simulink model "MtrCtrl_24V"  (R2023b)
settings: Solver=FixedStepDiscrete  StartTime=0.0  StopTime=1  FixedStep=1e-6  RelTol=1e-3
values from neighbouring files (symbols this model uses):
  B = 0.001889    [MtrCtrl_v01.sldd]    (also in PICal.m = 0.001889; PMSM.m = Simulink.Parameter)
  C_LUT_AngleTable_sng_Null = saveVarsMat.C_LUT_AngleTable_sng_Null    [AngleTable.m]    (also in MtrCtrl_v01.sldd = 0.0015339807878856412 0.0030679615757712823 0.00460194236365; PMSM.m; SinLut.m = sinTable(2,:))
  C_LUT_SinTable_sng_Null = saveVarsMat.C_LUT_SinTable_sng_Null    [AngleTable.m]    (also in MtrCtrl_v01.sldd = 0.0015339801862847655 0.0030679567629659761 0.00460192612044; PMSM.m; SinLut.m = sinTable(1,:))
  C_MATH_OneOverSqrtThree_s32n31_Null = 0.57735026918962584    [MtrCtrl_v01.sldd]    (also in PMSM.m = Simulink.Parameter)
  C_MATH_Pi_u32n30_Null = 3.1415926535897931    [MtrCtrl_v01.sldd]    (also in PMSM.m = Simulink.Parameter)
  C_MATH_SqrtThreeOverThree_s32n31_Null = 0.57735026918962573    [MtrCtrl_v01.sldd]    (also in PMSM.m = Simulink.Parameter)
  C_PMSM_CurQKi_u32n31_null = 0.15707963267949    [MtrCtrl_v01.sldd]    (also in PMSM.m = Simulink.Parameter)
  C_PMSM_CurQKp_u32n31_null = 19.949113350295185    [MtrCtrl_v01.sldd]    (also in PMSM.m = Simulink.Parameter)
  C_PMSM_Flux_u32n32_Vs = 0.192    [MtrCtrl_v01.sldd]    (also in PMSM.m = Simulink.Parameter)
  C_PMSM_Ls_pu = 0.398982267005904    [MtrCtrl_v01.sldd]
  C_PMSM_PolePairs_u8_Null = 4.0    [MtrCtrl_v01.sldd]
  Flux = 0.192    [MtrCtrl_v01.sldd]    (also in PICal.m; PMSM.m)
  IBase_A = 2000.0    [MtrCtrl_v01.sldd]    (also in PICal.m = 300; PMSM.m = Simulink.Parameter)
  J = 0.011    [MtrCtrl_v01.sldd]    (also in PICal.m; PMSM.m)
  K_CCM_MRASEna_bool_Flg = 0.0    [MtrCtrl_v01.sldd]
  K_SVM_DefultDuty_s32n31_Null = 0.25    [MtrCtrl_v01.sldd]    (also in PMSM.m = Simulink.Parameter)
  KCCM_VirPosn_flg = 0.0    [MtrCtrl_v01.sldd]    (also in PMSM.m = Simulink.Parameter)
  KCCM_VoltModeEna_Flg = 0.0    [MtrCtrl_v01.sldd]    (also in PMSM.m = Simulink.Parameter)
  Kis = 114583.3333333333    [MtrCtrl_v01.sldd]    (also in PICal.m = 114583.333333; PMSM.m = 114583.333333)
  KSMO_EnaEst_Flg = 0.0    [MtrCtrl_v01.sldd]    (also in PMSM.m = Simulink.Parameter)
  Kt = 1.1520000000000001    [MtrCtrl_v01.sldd]    (also in PICal.m = 1.152; PMSM.m = 1.152)
  Ld = 80e-6    (= 8e-05)    [FluxweakingGen.m]    (also in IEHB_MAPGenerationtest.m = 6.8e-05; MtrCtrl_v01.sldd = 0.000635
                
                    
             ; PICal.m = 0.000635; PMSM.m = Simulink.Parameter)
  LPF_coefg = 0.01    [MtrCtrl_v01.sldd]    (also in PMSM.m = Simulink.Parameter)
  Lq = 80e-6    (= 8e-05)    [FluxweakingGen.m]    (also in IEHB_MAPGenerationtest.m = 6e-05; MtrCtrl_v01.sldd = 0.000685
                
                    
             ; PICal.m = 0.000635; PMSM.m = Simulink.Parameter)
  Ls = 0.000635    [MtrCtrl_v01.sldd]    (also in PICal.m; PMSM.m)
  OneOverUBase_V = 0.0016666666666666668    [MtrCtrl_v01.sldd]    (also in PMSM.m = Simulink.Parameter)
  Pp = 4.0    [MtrCtrl_v01.sldd]    (also in PICal.m = 4; PMSM.m = Simulink.Parameter)
  Rs = 0.03    [FluxweakingGen.m]    (also in MtrCtrl_v01.sldd = 0.05
                
                    
                 ; PICal.m = 0.05; PMSM.m = Simulink.Parameter)
  SecPerRnd = 0.6    [MtrCtrl_v01.sldd]    (also in PMSM.m = Simulink.Parameter)
  sinTable = zeros(2,TableSize)    [SinLut.m]
  SMOGain_V = 323.31615074619043    [MtrCtrl_v01.sldd]    (also in PMSM.m = Simulink.Parameter)
  Ts = 1.0E-6    [MtrCtrl_v01.sldd]    (also in PICal.m = 0.0001; PMSM.m = Simulink.Parameter)
  TsCtrl = 1.0E-6    [MtrCtrl_v01.sldd]
  UBase_V = 600.0    [MtrCtrl_v01.sldd]    (also in PICal.m = 600; PMSM.m = Simulink.Parameter)
  wmBase_rps = 314.15926535897933    [MtrCtrl_v01.sldd]    (also in PICal.m = 314.159265359; PMSM.m = Simulink.Parameter)
undefined symbols (not defined in the file or in its folder): DiscIntNeverNeededParam, Ion, Lithium
libraries: ee_lib x16, spsVoltageMeasurementLib x14, simulink x11, spsSeriesRLCBranchLib x6, spsMosfetLib x6, nesl_utility x6, slpidlib x5, spsCurrentMeasurementLib x4, spsParallelRLCBranchLib x3, simulink_extras x2, spspowerguiLib x2, eePmsmFwController x1
(part 3 of 5)

== system MtrCtrl_24V/CurLpCtrl/Subsystem5 ==
  ParkPosn : Inport  OutDataTypeStr=fixdt(1,32,28)
  1-D Lookup Table : Lookup_n-D  NumberOfTableDimensions=1  BreakpointsForDimension1=C_LUT_AngleTable_sng_Null  BeginIndexSearchUsingPreviousIndexResult=on  Table=C_LUT_SinTable_sng_Null  ExtrapMethod=Clip  UseLastTableValue=on  ApplyFullPrecisionForLinearInterpolation=on  InternalRulePriority=Speed  OutDataTypeStr=fixdt(0,32,31)  RndMeth=Simplest
  1-D Lookup Table1 : Lookup_n-D  NumberOfTableDimensions=1  BreakpointsForDimension1=C_LUT_AngleTable_sng_Null  BeginIndexSearchUsingPreviousIndexResult=on  Table=C_LUT_SinTable_sng_Null  ExtrapMethod=Clip  UseLastTableValue=on  ApplyFullPrecisionForLinearInterpolation=on  InternalRulePriority=Speed  OutDataTypeStr=fixdt(0,32,31)  RndMeth=Simplest
  Add : Sum  OutDataTypeStr=fixdt(1,32,26)
  Chart : Stateflow chart  TreatAsAtomicUnit=on
  Constant1 : Constant  Value=0  OutDataTypeStr=fixdt(1,32,4)
  Gain : Gain  Gain=4  OutDataTypeStr=fixdt(1,32,26)
  Product : Product  OutDataTypeStr=fixdt(1,32,30)  RndMeth=Simplest
  Product1 : Product  OutDataTypeStr=fixdt(1,32,30)
  Scope : Scope  NumInputPorts=3
  SinTheta : Outport
  CosTheta : Outport  Port=2
  wires:
  ParkPosn/1 -> Gain/1
  Gain/1 -> Add/2
  Constant1/1 -> Add/1
  Product/1 -> Scope/1, SinTheta/1
  Product1/1 -> Scope/2, CosTheta/1
  Add/1 -> Scope/3, Chart/1(Angle)
  Chart/1(SinAngle) -> 1-D Lookup Table/1
  Chart/3(CosAngle) -> 1-D Lookup Table1/1
  1-D Lookup Table/1 -> Product/1
  Chart/2(SinSign) -> Product/2
  1-D Lookup Table1/1 -> Product1/1
  Chart/4(CosSign) -> Product1/2

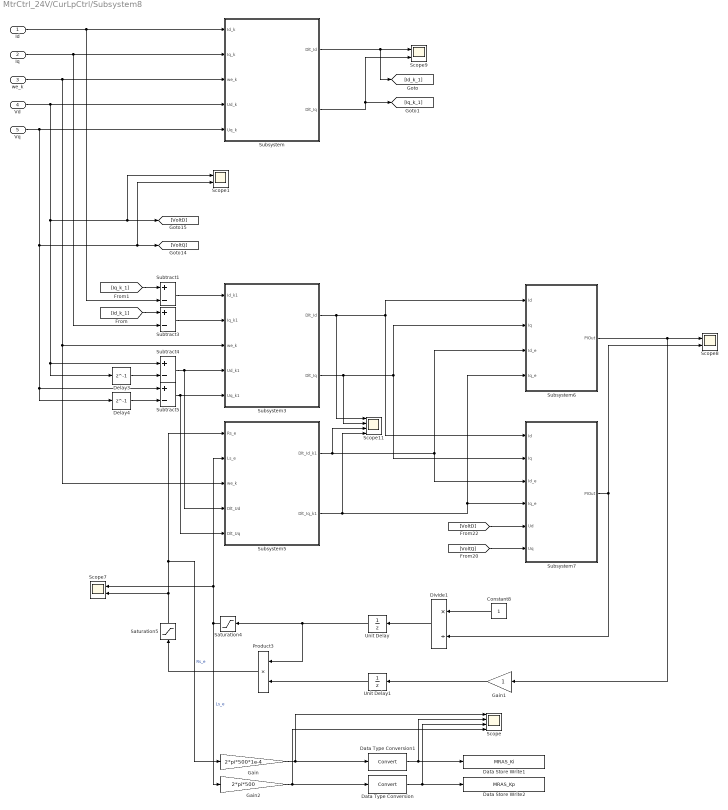
== system MtrCtrl_24V/CurLpCtrl/Subsystem8 ==
  Id : Inport
  Iq : Inport  Port=2
  we_k : Inport  Port=3
  Vd : Inport  Port=4
  Vq : Inport  Port=5
  Constant8 : Constant
  Data Store Write1 : DataStoreWrite  DataStoreName=MRAS_Ki  IndexOptions=Index vector (dialog)  Indices=1  OutputSizes=1
  Data Store Write2 : DataStoreWrite  DataStoreName=MRAS_Kp  IndexOptions=Index vector (dialog)  Indices=1  OutputSizes=1
  Data Type Conversion : DataTypeConversion  SaturateOnIntegerOverflow=off  RndMeth=Floor
  Data Type Conversion1 : DataTypeConversion  SaturateOnIntegerOverflow=off  RndMeth=Floor
  Delay3 : Delay  DelayLength=1
  Delay4 : Delay  DelayLength=1
  Divide1 : Product  Inputs=*/
  Gain : Gain  Gain=2*pi*500*1e-4
  Gain1 : Gain
  Gain2 : Gain  Gain=2*pi*500
  Product3 : Product
  Saturation4 : Saturate  UpperLimit=2*Ls  LowerLimit=1e-6
  Saturation5 : Saturate  UpperLimit=1.5*Rs  LowerLimit=1e-6
  Scope : Scope  NumInputPorts=4
  Scope{1,7..9} (4 alike) : Scope  NumInputPorts=2
  Scope11 : Scope  NumInputPorts=4
  Subsystem : Subsystem
  Subsystem3 : Subsystem
  Subsystem5 : Subsystem
  Subsystem6 : Subsystem
  Subsystem7 : Subsystem
  Subtract{1,3..5} (4 alike) : Sum  Inputs=+-
  Unit Delay : UnitDelay  SampleTime=-1  HasFrameUpgradeWarning=on
  Unit Delay1 : UnitDelay  SampleTime=-1  HasFrameUpgradeWarning=on
  wires:
  Subsystem/1(Dlt_Id) -> [Id_k_1], Scope9/1
  Delay3/1 -> Subtract4/2
  Subsystem3/1(Dlt_Id) -> Scope11/1, Subsystem6/1(Id), Subsystem7/1(Id)
  Subsystem5/2(Dlt_Iq_k1) -> Scope11/4, Subsystem7/4(Iq_e), Subsystem6/4(Iq_e)
  Subsystem5/1(Dlt_Id_k1) -> Scope11/3, Subsystem6/3(Id_e), Subsystem7/3(Id_e)
  we_k/1 -> Subsystem5/3(we_k), Subsystem3/3(we_k), Subsystem/3(we_k)
  Subtract4/1 -> Subsystem5/4(Dlt_Ud), Subsystem3/4(Ud_k1)
  Id/1 -> Subsystem/1(Id_k), Subtract1/2
  [VoltD] -> Subsystem7/5(Ud)
  Vq/1 -> Scope1/2, [VoltQ], Delay4/1, Subtract5/1, Subsystem/5(Uq_k)
  Subtract5/1 -> Subsystem5/5(Dlt_Uq), Subsystem3/5(Uq_k1)
  Iq/1 -> Subtract3/2, Subsystem/2(Iq_k)
  Subsystem3/2(Dlt_Iq) -> Scope11/2, Subsystem7/2(Iq), Subsystem6/2(Iq)
  Saturation5/1 -> Gain/1, Subsystem5/1(Rs_e), Scope7/2  "Rs_e"
  [VoltQ] -> Subsystem7/6(Uq)
  Constant8/1 -> Divide1/1
  Gain/1 -> Scope/1, Data Type Conversion1/1
  Saturation4/1 -> Subsystem5/2(Ls_e), Scope7/1, Gain2/1  "Ls_e"
  Subtract3/1 -> Subsystem3/2(Iq_k1)
  Subsystem/2(Dlt_Iq) -> [Iq_k_1], Scope9/2
  Subtract1/1 -> Subsystem3/1(Id_k1)
  Delay4/1 -> Subtract5/2
  Divide1/1 -> Unit Delay/1
  Subsystem7/1(PIOut) -> Divide1/2, Scope8/2
  Unit Delay1/1 -> Product3/2
  Product3/1 -> Saturation5/1
  Unit Delay/1 -> Product3/1, Saturation4/1
  Vd/1 -> Scope1/1, [VoltD], Delay3/1, Subtract4/1, Subsystem/4(Ud_k)
  Gain2/1 -> Scope/4, Data Type Conversion/1
  Data Type Conversion/1 -> Scope/3, Data Store Write2/1
  Data Type Conversion1/1 -> Scope/2, Data Store Write1/1
  [Iq_k_1] -> Subtract1/1
  [Id_k_1] -> Subtract3/1
  Subsystem6/1(PIOut) -> Gain1/1, Scope8/1
  Gain1/1 -> Unit Delay1/1

== system MtrCtrl_24V/CurLpCtrl/VDQLimit ==
  VdCmd : Inport  OutDataTypeStr=fixdt(1,32,31)
  VqCmd : Inport  Port=2  OutDataTypeStr=fixdt(1,32,31)
  Udc : Inport  Port=3  OutDataTypeStr=fixdt(0,32,32)
  Add : Sum  OutDataTypeStr=fixdt(0,32,32)
  Compare To Constant : simulink/Logic and Bit Operations/Compare To Constant  relop=>=  const=1  OutDataTypeStr=boolean
  Demux1 : Demux  Outputs=2
  Divide : Product  Inputs=/*  OutDataTypeStr=fixdt(0,32,21)
  Gain : Gain  Gain=0.91  OutDataTypeStr=fixdt(0,32,32)
  Mux : Mux  Inputs=2
  Mux1 : Mux  Inputs=2
  Product : Product  OutDataTypeStr=fixdt(0,32,35)
  Product1 : Product  OutDataTypeStr=fixdt(0,32,33)
  Product2 : Product  OutDataTypeStr=fixdt(1,32,31)
  Product3 : Product  OutDataTypeStr=fixdt(1,32,31)
  Scope : Scope  NumInputPorts=3
  Scope1 : Scope
  Scope2 : Scope
  Scope3 : Scope  NumInputPorts=2
  Sqrt : Sqrt  OutDataTypeStr=fixdt(0,32,32)
  Switch : Switch  Criteria=u2 ~= 0  Threshold=1  OutDataTypeStr=fixdt(1,32,31)  SaturateOnIntegerOverflow=off  InputSameDT=off
  VdCmd1 : InportShadow  OutDataTypeStr=fixdt(1,32,31)
  VqCmd1 : InportShadow  Port=2  OutDataTypeStr=fixdt(1,32,31)
  VdLimit : Outport
  VqLimit : Outport  Port=2
  wires:
  VdCmd/1 -> Product2/2, Product/2, Product/1
  Product/1 -> Add/1
  VqCmd/1 -> Product1/2, Product3/2, Product1/1
  Product1/1 -> Add/2
  Add/1 -> Scope2/1, Sqrt/1
  Sqrt/1 -> Divide/1
  Udc/1 -> Gain/1
  Divide/1 -> Scope/3, Compare To Constant/1, Product2/1, Product3/1  "Kv"
  Compare To Constant/1 -> Scope1/1, Switch/2
  VdCmd1/1 -> Mux/1
  VqCmd1/1 -> Mux/2
  Mux/1 -> Switch/1
  Product2/1 -> Scope/2, Mux1/1  "VdLimit"
  Product3/1 -> Scope/1, Mux1/2  "VqLimit"
  Mux1/1 -> Switch/3
  Switch/1 -> Demux1/1
  Demux1/1 -> Scope3/1, VdLimit/1
  Demux1/2 -> Scope3/2, VqLimit/1
  Gain/1 -> Divide/2

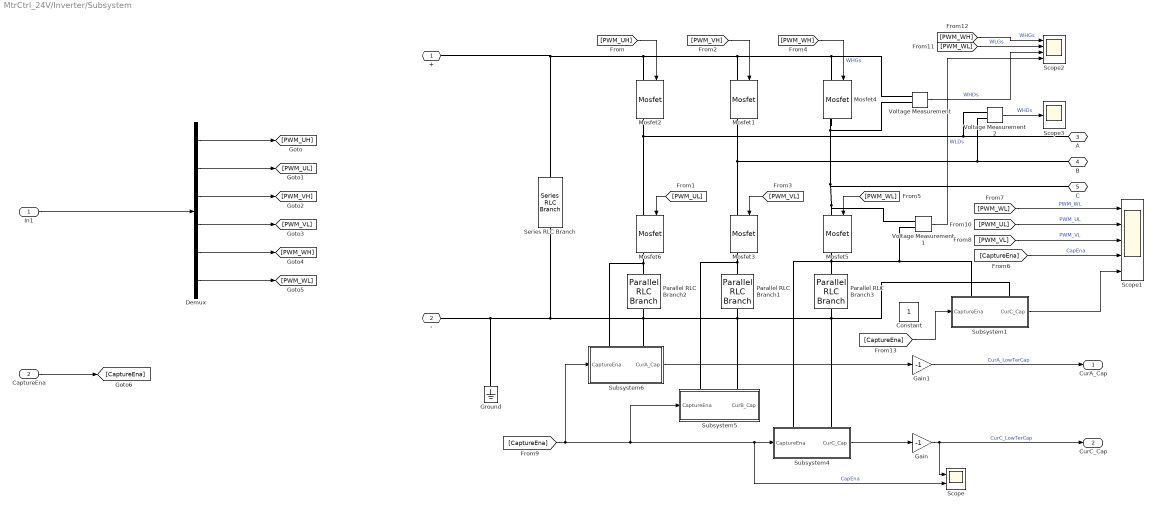
== system MtrCtrl_24V/Inverter/Subsystem ==
  In1 : Inport
  CaptureEna : Inport  Port=2
  Constant : Constant
  Demux : Demux  Outputs=6
  Gain : Gain  Gain=-1
  Gain1 : Gain  Gain=-1
  Ground : spsGroundLib/Ground  LConnTagsString=a
  Mosfet{1..6} (6 alike) : spsMosfetLib/Mosfet  Ron=0.0005  Lon=0  Rd=0.001  Vfd=0  IC=0  Rs=1e5  Cs=inf  Measurements=on
  Parallel RLC Branch1 : spsParallelRLCBranchLib/Parallel RLC Branch  LConnTagsString=a  RConnTagsString=__new0  BranchType=RC  Resistance=0.001  Inductance=1e-5  SetiL0=off  InitialCurrent=0  Capacitance=47e-9  Setx0=off  InitialVoltage=0  Measurements=None
  Parallel RLC Branch2 : spsParallelRLCBranchLib/Parallel RLC Branch  LConnTagsString=a  RConnTagsString=__new0  BranchType=RC  Resistance=0.001  Inductance=1e-5  SetiL0=off  InitialCurrent=0  Capacitance=47e-9  Setx0=off  InitialVoltage=0  Measurements=None
  Parallel RLC Branch3 : spsParallelRLCBranchLib/Parallel RLC Branch  LConnTagsString=a  RConnTagsString=__new0  BranchType=RC  Resistance=0.001  Inductance=1e-5  SetiL0=off  InitialCurrent=0  Capacitance=47e-9  Setx0=off  InitialVoltage=0  Measurements=None
  Scope : Scope  NumInputPorts=2
  Scope1 : Scope  NumInputPorts=5
  Scope2 : Scope  NumInputPorts=4
  Scope3 : Scope
  Series RLC Branch : spsSeriesRLCBranchLib/Series RLC Branch  LConnTagsString=__new0  RConnTagsString=__new0  BranchType=RC  Resistance=0.01  Inductance=1e-3  SetiL0=off  InitialCurrent=0  Capacitance=3e-3  Setx0=off  InitialVoltage=0  Measurements=None
  Subsystem1 : Subsystem
      settings: PortSchema="{\"entries\":[{\"content\":{\"sides\":[{\"content\":{\"connectorIds\":[\"LConn1\",\"LConn2\"]},\"type\":\"ConnectorPlacement.EquallySpacedRectSide\",\"uuid\":\"96a0a102-57f3-4e2a-918e-d16313977653\"},{\"content\":{\"connectorIds\":[],\"side\":\"RIGHT\"},\"type\":\"ConnectorPlacement.EquallySpacedRectSide\",\"uuid\":\"a5f84fe1-144b-47e8-bcf4-8bb651666773\"},{\"content\":{\"connectorIds\":[\"Out1\"],\"side\":\"TOP\"},\"type\":\"ConnectorPlacement.EquallySpacedRectSide\",\"uuid\":\"8129e7a0-5870-4724-806c-9a69f94ba6e8\"},{\"content\":{\"connectorIds\":[\"In1\"],\"side\":\"BOTTOM\"},\"type\":\"ConnectorPlacement.EquallySpacedRectSide\",\"uuid\":\"c5913083-b261-46af-9138-fed3dfb04ce1\"}]},\"type\":\"ConnectorPlacement.EquallySpacedConnector\",\"uuid\":\"44cbcd78-856c-4eaa-a248-411ae20b5f24\"}],\"packageUris\":[\"http://schema.mathworks.com/mf0/Connector/R2020b\"],\"version\":\"1.0\"}"
  Subsystem4 : Subsystem
      settings: PortSchema="{\"entries\":[{\"content\":{\"sides\":[{\"content\":{\"connectorIds\":[\"LConn1\",\"LConn2\"]},\"type\":\"ConnectorPlacement.EquallySpacedRectSide\",\"uuid\":\"96a0a102-57f3-4e2a-918e-d16313977653\"},{\"content\":{\"connectorIds\":[],\"side\":\"RIGHT\"},\"type\":\"ConnectorPlacement.EquallySpacedRectSide\",\"uuid\":\"a5f84fe1-144b-47e8-bcf4-8bb651666773\"},{\"content\":{\"connectorIds\":[\"Out1\"],\"side\":\"TOP\"},\"type\":\"ConnectorPlacement.EquallySpacedRectSide\",\"uuid\":\"8129e7a0-5870-4724-806c-9a69f94ba6e8\"},{\"content\":{\"connectorIds\":[\"In1\"],\"side\":\"BOTTOM\"},\"type\":\"ConnectorPlacement.EquallySpacedRectSide\",\"uuid\":\"c5913083-b261-46af-9138-fed3dfb04ce1\"}]},\"type\":\"ConnectorPlacement.EquallySpacedConnector\",\"uuid\":\"44cbcd78-856c-4eaa-a248-411ae20b5f24\"}],\"packageUris\":[\"http://schema.mathworks.com/mf0/Connector/R2020b\"],\"version\":\"1.0\"}"
  Subsystem5 : Subsystem
      settings: PortSchema="{\"entries\":[{\"content\":{\"sides\":[{\"content\":{\"connectorIds\":[\"LConn1\",\"LConn2\"]},\"type\":\"ConnectorPlacement.EquallySpacedRectSide\",\"uuid\":\"96a0a102-57f3-4e2a-918e-d16313977653\"},{\"content\":{\"connectorIds\":[],\"side\":\"RIGHT\"},\"type\":\"ConnectorPlacement.EquallySpacedRectSide\",\"uuid\":\"a5f84fe1-144b-47e8-bcf4-8bb651666773\"},{\"content\":{\"connectorIds\":[\"Out1\"],\"side\":\"TOP\"},\"type\":\"ConnectorPlacement.EquallySpacedRectSide\",\"uuid\":\"8129e7a0-5870-4724-806c-9a69f94ba6e8\"},{\"content\":{\"connectorIds\":[\"In1\"],\"side\":\"BOTTOM\"},\"type\":\"ConnectorPlacement.EquallySpacedRectSide\",\"uuid\":\"c5913083-b261-46af-9138-fed3dfb04ce1\"}]},\"type\":\"ConnectorPlacement.EquallySpacedConnector\",\"uuid\":\"44cbcd78-856c-4eaa-a248-411ae20b5f24\"}],\"packageUris\":[\"http://schema.mathworks.com/mf0/Connector/R2020b\"],\"version\":\"1.0\"}"
  Subsystem6 : Subsystem
      settings: PortSchema="{\"entries\":[{\"content\":{\"sides\":[{\"content\":{\"connectorIds\":[\"LConn1\",\"LConn2\"]},\"type\":\"ConnectorPlacement.EquallySpacedRectSide\",\"uuid\":\"96a0a102-57f3-4e2a-918e-d16313977653\"},{\"content\":{\"connectorIds\":[],\"side\":\"RIGHT\"},\"type\":\"ConnectorPlacement.EquallySpacedRectSide\",\"uuid\":\"a5f84fe1-144b-47e8-bcf4-8bb651666773\"},{\"content\":{\"connectorIds\":[\"Out1\"],\"side\":\"TOP\"},\"type\":\"ConnectorPlacement.EquallySpacedRectSide\",\"uuid\":\"8129e7a0-5870-4724-806c-9a69f94ba6e8\"},{\"content\":{\"connectorIds\":[\"In1\"],\"side\":\"BOTTOM\"},\"type\":\"ConnectorPlacement.EquallySpacedRectSide\",\"uuid\":\"c5913083-b261-46af-9138-fed3dfb04ce1\"}]},\"type\":\"ConnectorPlacement.EquallySpacedConnector\",\"uuid\":\"44cbcd78-856c-4eaa-a248-411ae20b5f24\"}],\"packageUris\":[\"http://schema.mathworks.com/mf0/Connector/R2020b\"],\"version\":\"1.0\"}"
  Voltage Measurement : spsVoltageMeasurementLib/Voltage Measurement  PhasorSimulation=off  OutputType=Complex  PSBequivalent=0
  Voltage Measurement1 : spsVoltageMeasurementLib/Voltage Measurement  PhasorSimulation=off  OutputType=Complex  PSBequivalent=0
  Voltage Measurement2 : spsVoltageMeasurementLib/Voltage Measurement  PhasorSimulation=off  OutputType=Complex  PSBequivalent=0
  + : PMIOPort  Side=Left
  - : PMIOPort  Port=2  Side=Left
  A : PMIOPort  Port=3  Side=Right
  B : PMIOPort  Port=4  Side=Right
  C : PMIOPort  Port=5  Side=Right
  CurA_Cap : Outport
  CurC_Cap : Outport  Port=2
  wires:
  Demux/1 -> [PWM_UH]
  In1/1 -> Demux/1
  [PWM_UH] -> Mosfet2/1
  Demux/2 -> [PWM_UL]
  [PWM_UL] -> Mosfet6/1
  Demux/3 -> [PWM_VH]
  Demux/4 -> [PWM_VL]
  Demux/5 -> [PWM_WH]
  [PWM_VH] -> Mosfet1/1
  Demux/6 -> [PWM_WL]
  [PWM_VL] -> Mosfet3/1
  [PWM_WH] -> Mosfet4/1  "WHGs"
  [PWM_WL] -> Mosfet5/1
  CaptureEna/1 -> [CaptureEna]
  [CaptureEna] -> Subsystem6/1(CaptureEna), Subsystem5/1(CaptureEna), Scope/2, Subsystem4/1(CaptureEna)  "CapEna"
  Subsystem6/1(CurA_Cap) -> Gain1/1
  Subsystem4/1(CurC_Cap) -> Gain/1
  Gain1/1 -> CurA_Cap/1  "CurA_LowTerCap"
  Gain/1 -> Scope/1, CurC_Cap/1  "CurC_LowTerCap"
  [CaptureEna] -> Scope1/4  "CapEna"
  [CaptureEna] -> Subsystem1/1(CaptureEna)
  [PWM_WL] -> Scope1/1  "PWM_WL"
  [PWM_VL] -> Scope1/3  "PWM_VL"
  [PWM_UL] -> Scope1/2  "PWM_UL"
  Subsystem1/1(CurC_Cap) -> Scope1/5
  Voltage Measurement/1 -> Scope2/3  "WHDs"
  Voltage Measurement1/1 -> Scope2/4  "WLDs"
  [PWM_WL] -> Scope2/2  "WLGs"
  [PWM_WH] -> Scope2/1  "WHGs"
  Voltage Measurement2/1 -> Scope3/1  "WHDs"
  connections:
  Voltage Measurement2/LConn1 -- A/RConn1 -- Mosfet6/LConn1 -- Mosfet2/RConn1
  Parallel RLC Branch2/LConn1 -- Mosfet6/RConn1 -- Subsystem6/LConn2
  Mosfet4/LConn1 -- Voltage Measurement/LConn1 -- Mosfet1/LConn1 -- Mosfet2/LConn1 -- Series RLC Branch/LConn1 -- +/RConn1
  Mosfet5/RConn1 -- Subsystem1/LConn2 -- Voltage Measurement1/LConn2 -- Parallel RLC Branch3/LConn1 -- Subsystem4/LConn2
  Mosfet3/RConn1 -- Parallel RLC Branch1/LConn1 -- Subsystem5/LConn2
  Parallel RLC Branch1/RConn1 -- Subsystem5/LConn1 -- Subsystem4/LConn1 -- Parallel RLC Branch3/RConn1 -- Subsystem1/LConn1 -- Subsystem6/LConn1 -- Parallel RLC Branch2/RConn1 -- Series RLC Branch/RConn1 -- -/RConn1 -- Ground/LConn1
  Mosfet5/LConn1 -- Voltage Measurement/LConn2 -- Mosfet4/RConn1 -- C/RConn1 -- Voltage Measurement1/LConn1
  Voltage Measurement2/LConn2 -- B/RConn1 -- Mosfet3/LConn1 -- Mosfet1/RConn1

== system MtrCtrl_24V/MotorModel/Subsystem ==
  TLoad : Inport
  Va : Inport  Port=2
  Vb : Inport  Port=3
  Vc : Inport  Port=4
  Theta_In : Inport  Port=5
  Bus Creator : BusCreator  Inputs=5
  ClarkeTF : Subsystem
  InversePark : Subsystem
  ParkTF : Subsystem
  Scope : Scope  NumInputPorts=2
  Scope1 : Scope  NumInputPorts=2
  Scope2 : Scope  NumInputPorts=3
  Scope4 : Scope  NumInputPorts=2
  Subsystem : Subsystem
  Subsystem1 : Subsystem
  Subsystem2 : Subsystem
  Subsystem3 : Subsystem
  Te : Outport
  wm : Outport  Port=2
  Speed_rpm : Outport  Port=3
  theta : Outport  Port=4
  CurMaesure : Outport  Port=5
  wires:
  Va/1 -> Scope2/1, ClarkeTF/1(Va)
  Vb/1 -> Scope2/2, ClarkeTF/2(Vb)
  ClarkeTF/1(V_alpha) -> Scope4/1, ParkTF/1(Valpha)
  ClarkeTF/2(V_beta) -> Scope4/2, ParkTF/2(Vbeta)
  [SinTheta] -> Scope/1, ParkTF/3(SinTheta)
  [CosTheta] -> Scope/2, ParkTF/4(CosTheta)
  ParkTF/1(Vd) -> Scope1/1, Subsystem/1(Vd)  "Vd_V"
  ParkTF/2(Vq) -> Scope1/2, Subsystem/2(Vq)  "Vq_V"
  Subsystem/2(Iq) -> InversePark/2(Q), Bus Creator/5, Subsystem1/2(Iq)  "Iq"
  Subsystem/1(Id) -> InversePark/1(D), Bus Creator/4, Subsystem1/1(Id)  "Id"
  Subsystem1/5(we) -> Subsystem/3(we)
  Subsystem2/1(SinTheta) -> [SinTheta]
  Subsystem2/2(CoTheta) -> [CosTheta]
  TLoad/1 -> Subsystem1/3(TLoad)
  Subsystem1/1(Te) -> Te/1
  Subsystem1/2(wm) -> wm/1
  Subsystem1/3(Speed_rpm) -> Speed_rpm/1
  [SinTheta] -> InversePark/3(SinTheta)
  [CosTheta] -> InversePark/4(CosTheta)
  InversePark/1(Alpha) -> Subsystem3/1(Alpha)
  InversePark/2(Beta) -> Subsystem3/2(Beta)
  Subsystem3/1(CurA) -> Bus Creator/1  "CurA"
  Subsystem3/3(CurC) -> Bus Creator/3  "CurC"
  Subsystem3/2(CurB) -> Bus Creator/2  "CurB"
  Bus Creator/1 -> CurMaesure/1
  Subsystem1/4(theta) -> Subsystem2/2(Theta_Mtr), theta/1
  Theta_In/1 -> Subsystem2/1(Theta_In)
  Vc/1 -> Scope2/3

== system MtrCtrl_24V/SpdCtrl/Subsystem1 ==
  Ref : Inport
  Fbk : Inport  Port=2
  Sat : Inport  Port=3
  Add : Sum
  Add1 : Sum  Inputs=+++
  Add2 : Sum  Inputs=+-
  Add3 : Sum
  Gain : Gain  Gain=0.06
  Ki : Constant  Value=1/Kis
  Kp : Constant  Value=1.0
  Kp1 : Constant  Value=0
  Product : Product
  Product1 : Product
  Product2 : Product
  Relational Operator : RelationalOperator  Operator=<=  OutDataTypeStr=boolean  RndMeth=Simplest  InputSameDT=off
  Saturation : Saturate  UpperLimit=220  LowerLimit=-15
  Saturation1 : Saturate  UpperLimit=130  LowerLimit=-15
  Switch : Switch  Criteria=u2 > Threshold  SaturateOnIntegerOverflow=off  InputSameDT=off
  Unit Delay : UnitDelay  SampleTime=-1  HasFrameUpgradeWarning=on
  Unit Delay1 : UnitDelay  SampleTime=-1  HasFrameUpgradeWarning=on
  PIOut : Outport
  wires:
  Kp/1 -> Product/2
  Add1/1 -> PIOut/1
  Product/1 -> Saturation/1
  Add2/1 -> Unit Delay1/1, Add3/1, Product1/2, Product/1
  Add/1 -> Switch/1, Relational Operator/1
  Ki/1 -> Product1/1
  Relational Operator/1 -> Switch/2
  Gain/1 -> Relational Operator/2, Switch/3
  Sat/1 -> Gain/1
  Switch/1 -> Add1/2, Unit Delay/1
  Ref/1 -> Add2/1
  Fbk/1 -> Add2/2
  Saturation/1 -> Add1/1
  Product1/1 -> Add/1
  Unit Delay/1 -> Add/2
  Unit Delay1/1 -> Add3/2
  Add3/1 -> Product2/1
  Kp1/1 -> Product2/2
  Product2/1 -> Saturation1/1
  Saturation1/1 -> Add1/3

== system MtrCtrl_24V/Subsystem8/Subsystem ==
  Id_k : Inport
  Iq_k : Inport  Port=2
  we_k : Inport  Port=3
  Ud_k : Inport  Port=4
  Uq_k : Inport  Port=5
  Add2 : Sum
  Add3 : Sum
  Add4 : Sum
  Add5 : Sum  Inputs=+++
  Constant1 : Constant  Value=1-Ts*Rs/Ls
  Constant18 : Constant  Value=-Ts*Flux/Ls
  Constant2 : Constant  Value=Ts/Ls
  Constant3 : Constant  Value=1-Ts*Rs/Ls
  Constant4 : Constant  Value=Ts/Ls
  Gain6 : Gain  Gain=Ts
  Gain7 : Gain  Gain=-1
  Id_k_copy : InportShadow
  Iq_k_copy : InportShadow  Port=2
  Product{5,9..14} (7 alike) : Product
  Subtract : Sum  Inputs=+-
  Subtract1 : Sum  Inputs=+-
  Dlt_Id : Outport
  Dlt_Iq : Outport  Port=2
  wires:
  Product14/1 -> Add5/3
  Constant2/1 -> Product13/1
  Product10/1 -> Add3/1
  Gain6/1 -> Gain7/1, Product9/2
  Constant1/1 -> Product11/1
  Uq_k/1 -> Product13/2
  Product5/1 -> Add2/1
  Product9/1 -> Add2/2
  Product12/1 -> Add4/2
  Id_k/1 -> Product10/2, Product5/1
  Product11/1 -> Add3/2
  Constant4/1 -> Product12/1
  Add2/1 -> Add4/1
  Iq_k/1 -> Product11/2, Product9/1
  Constant18/1 -> Product14/1
  Add5/1 -> Subtract1/1  "Iq_k_1"
  we_k/1 -> Product14/2, Gain6/1
  Gain7/1 -> Product10/1
  Constant3/1 -> Product5/2
  Add3/1 -> Add5/1
  Add4/1 -> Subtract/1  "Id_k_1"
  Product13/1 -> Add5/2
  Ud_k/1 -> Product12/2
  Id_k_copy/1 -> Subtract/2
  Subtract/1 -> Dlt_Id/1
  Subtract1/1 -> Dlt_Iq/1
  Iq_k_copy/1 -> Subtract1/2

== system MtrCtrl_24V/Subsystem8/Subsystem3 ==
  Id_k1 : Inport
  Iq_k1 : Inport  Port=2
  we_k : Inport  Port=3
  Ud_k1 : Inport  Port=4
  Uq_k1 : Inport  Port=5
  Add2 : Sum
  Add3 : Sum
  Add4 : Sum
  Add5 : Sum  Inputs=+++
  Constant1 : Constant  Value=1-Ts*Rs/Ls
  Constant14 : Constant  Value=1-Ts*Rs/Ls
  Constant16 : Constant  Value=Ts/Ls
  Constant18 : Constant  Value=-Ts*Flux/Ls
  Constant2 : Constant  Value=Ts/Ls
  Gain6 : Gain  Gain=Ts
  Gain7 : Gain  Gain=-1
  Id_k1_Copy : InportShadow
  Iq_k1_Copy : InportShadow  Port=2
  Product{5,9..14} (7 alike) : Product
  Subtract : Sum  Inputs=+-
  Subtract1 : Sum  Inputs=+-
  Dlt_Id : Outport
  Dlt_Iq : Outport  Port=2
  wires:
  Iq_k1_Copy/1 -> Subtract1/2
  Subtract1/1 -> Dlt_Iq/1
  Subtract/1 -> Dlt_Id/1
  Id_k1_Copy/1 -> Subtract/2
  Ud_k1/1 -> Product12/2
  Product13/1 -> Add5/2
  Add4/1 -> Subtract/1  "Id_k2"
  Add3/1 -> Add5/1
  Constant14/1 -> Product5/2
  Gain7/1 -> Product10/1
  we_k/1 -> Gain6/1, Product14/2
  Add5/1 -> Subtract1/1  "Iq_k2"
  Constant18/1 -> Product14/1
  Iq_k1/1 -> Product9/1, Product11/2
  Add2/1 -> Add4/1
  Constant16/1 -> Product12/1
  Product11/1 -> Add3/2
  Id_k1/1 -> Product5/1, Product10/2
  Product12/1 -> Add4/2
  Product9/1 -> Add2/2
  Product5/1 -> Add2/1
  Uq_k1/1 -> Product13/2
  Constant1/1 -> Product11/1
  Gain6/1 -> Product9/2, Gain7/1
  Product10/1 -> Add3/1
  Constant2/1 -> Product13/1
  Product14/1 -> Add5/3

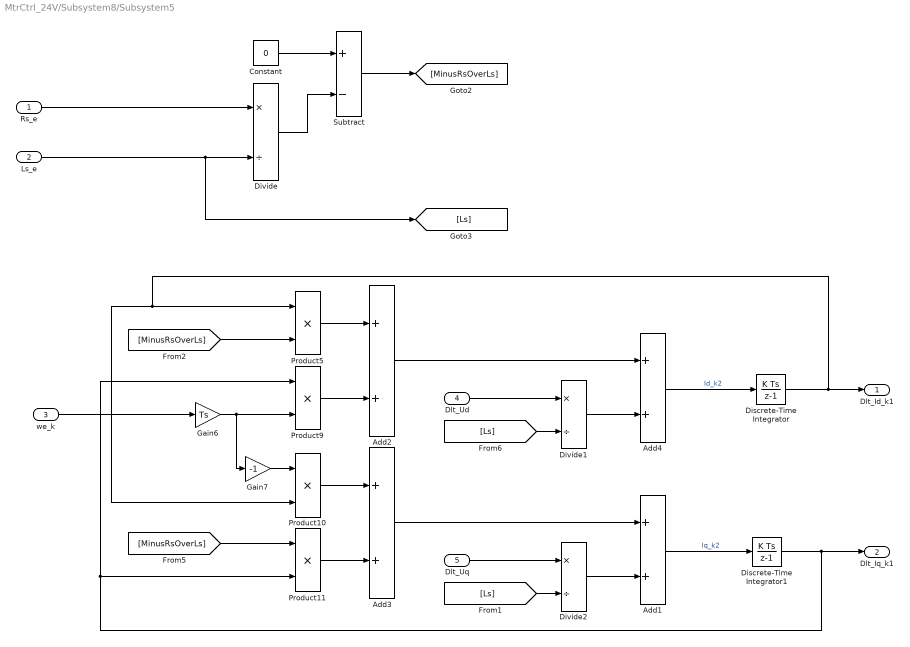
== system MtrCtrl_24V/Subsystem8/Subsystem5 ==
  Rs_e : Inport
  Ls_e : Inport  Port=2
  we_k : Inport  Port=3
  Dlt_Ud : Inport  Port=4
  Dlt_Uq : Inport  Port=5
  Add{1..4} (4 alike) : Sum
  Constant : Constant  Value=0
  Discrete-Time Integrator : DiscreteIntegrator  SampleTime=-1  ICPrevOutput=DiscIntNeverNeededParam  ICPrevScaledInput=DiscIntNeverNeededParam
  Discrete-Time Integrator1 : DiscreteIntegrator  SampleTime=-1  ICPrevOutput=DiscIntNeverNeededParam  ICPrevScaledInput=DiscIntNeverNeededParam
  Divide : Product  Inputs=*/
  Divide1 : Product  Inputs=*/
  Divide2 : Product  Inputs=*/
  Gain6 : Gain  Gain=Ts
  Gain7 : Gain  Gain=-1
  Product{5,9..11} (4 alike) : Product
  Subtract : Sum  Inputs=+-
  Dlt_Id_k1 : Outport
  Dlt_Iq_k1 : Outport  Port=2
  wires:
  Dlt_Ud/1 -> Divide1/1
  Divide2/1 -> Add1/2
  Add4/1 -> Discrete-Time Integrator/1  "Id_k2"
  Add3/1 -> Add1/1
  [MinusRsOverLs] -> Product5/2
  Gain7/1 -> Product10/1
  we_k/1 -> Gain6/1
  Add1/1 -> Discrete-Time Integrator1/1  "Iq_k2"
  Discrete-Time Integrator1/1 -> Dlt_Iq_k1/1, Product9/1, Product11/2
  Add2/1 -> Add4/1
  [Ls] -> Divide1/2
  Product11/1 -> Add3/2
  Discrete-Time Integrator/1 -> Product10/2, Product5/1, Dlt_Id_k1/1
  Divide1/1 -> Add4/2
  Product9/1 -> Add2/2
  Product5/1 -> Add2/1
  Dlt_Uq/1 -> Divide2/1
  [MinusRsOverLs] -> Product11/1
  Gain6/1 -> Product9/2, Gain7/1
  Product10/1 -> Add3/1
  Constant/1 -> Subtract/1
  Rs_e/1 -> Divide/1
  Divide/1 -> Subtract/2
  Subtract/1 -> [MinusRsOverLs]
  Ls_e/1 -> [Ls], Divide/2
  [Ls] -> Divide2/2

== system MtrCtrl_24V/Subsystem8/Subsystem6 ==
  Id : Inport
  Iq : Inport  Port=2
  Id_e : Inport  Port=3
  Iq_e : Inport  Port=4
  Abs : Abs  SaturateOnIntegerOverflow=off
  Add : Sum
  Constant2 : Constant  Value=0.5
  Constant3 : Constant  Value=0.002
  Constant8 : Constant  Commented=on  Value=2*Rs/Ls
  PID Controller : slpidlib/PID Controller  Controller=PI  Form=Parallel  TimeDomain=Discrete-time  UseExternalTs=off  SampleTime=-1  IntegratorMethod=Forward Euler  FilterMethod=Forward Euler  ControllerParametersSource=external  P=1  I=1  UseKiTs=off  D=0  N=100  UseFilter=on  TunerSelectOption=Transfer Function Based (PID Tuner App)  InitialConditionSource=internal  InitialConditionForIntegrator=0  InitialConditionForFilter=0  DifferentiatorICPrevScaledInput=0  ExternalReset=none  TrackingMode=off  Kt=1  LimitOutput=off  SatLimitsSource=internal  UpperSaturationLimit=inf  LowerSaturationLimit=-inf  LinearizeAsGain=on  AntiWindupMode=none  Kb=1  LimitIntegrator=off  UpperIntegratorSaturationLimit=inf  LowerIntegratorSaturationLimit=-inf  POutMin=[]  POutMax=[]  IOutMin=[]  IOutMax=[]  DOutMin=[]  DOutMax=[]  NOutMin=[]  NOutMax=[]  SumOutMin=[]  SumOutMax=[]  SaturationOutMin=[]  SaturationOutMax=[]  PParamMin=[]  PParamMax=[]  IParamMin=[]  IParamMax=[]  DParamMin=[]  DParamMax=[]  NParamMin=[]  NParamMax=[]  KbParamMin=[]  KbParamMax=[]  KtParamMin=[]  KtParamMax=[]  KbOutMin=[]  KbOutMax=[]  KtOutMin=[]  KtOutMax=[]  IntegratorOutMin=[]  IntegratorOutMax=[]  FilterOutMin=[]  FilterOutMax=[]  SumI1OutMin=[]  SumI1OutMax=[]  SumI2OutMin=[]  SumI2OutMax=[]  SumI3OutMin=[]  SumI3OutMax=[]  SumI4OutMin=[]  SumI4OutMax=[]  SumDOutMin=[]  SumDOutMax=[]  DifferentiatorOutMin=[]  DifferentiatorOutMax=[]  FilterDiffOutCoefMin=[]  FilterDiffOutCoefMax=[]  ReciprocalOutMin=[]  ReciprocalOutMax=[]  SumDenOutMin=[]  SumDenOutMax=[]  SumNumOutMin=[]  SumNumOutMax=[]  DivideOutMin=[]  DivideOutMax=[]  UdiffTsProdOutMin=[]  UdiffTsProdOutMax=[]  NTsProdOutMin=[]  NTsProdOutMax=[]  UintegralTsProdOutMin=[]  UintegralTsProdOutMax=[]  UngainTsProdOutMin=[]  UngainTsProdOutMax=[]  ClampingZeroOutDataTypeStr=Inherit: Inherit via back propagation  ClampingZeroOutMin=[]  ClampingZeroOutMax=[]  FilterDenConstantOutDataTypeStr=Inherit: Inherit via back propagation  FilterDenConstantOutMin=[]  FilterDenConstantOutMax=[]  PCopyOutDataTypeStr=Inherit: Inherit via back propagation  PCopyOutMin=[]  PCopyOutMax=[]  NCopyOutDataTypeStr=Inherit: Inherit via back propagation  NCopyOutMin=[]  NCopyOutMax=[]  IntegratorContinuousStateAttributes=''  IntegratorStateMustResolveToSignalObject=off  IntegratorRTWStateStorageClass=Auto  FilterContinuousStateAttributes=''  FilterStateMustResolveToSignalObject=off  FilterRTWStateStorageClass=Auto  ParallelPVariant=ExternalParameters  IdealPVariant=Disabled  IVariant=ExternalParameters  DVariant=Disabled  IntegratorVariant=Discrete  SatVariant=Disabled  AWVariant=Passthrough  PCopyVariant=Disabled  TRVariant=Disabled  FdbkBlocksVariant=Forward  IdealPFdbkVariant=Disabled  SatFdbkVariant=Disabled  DerivativeFilterVariant=Disabled  NVariant=Disabled  NCopyVariant=Disabled_SignalSpec  FilterICVariant=Disabled  IntegratorICVariant=InternalICs  ExternalResetVariant=Disabled  TRSumVariant=Passthrough  SumFdbkVariant=Disabled  SumVariant=Sum_PI  TsampFilterVariant=InternalTs  TsampNgainVariant=Passthrough  TsampIntegralVariant=Disabled_SignalSpec  ExternalSaturationOutDataTypeStr=Inherit: Same as second input
  Product3 : Product
  Product5 : Product
  Saturation : Saturate  UpperLimit=20*Rs/Ls  LowerLimit=1e-6
  Subtract6 : Sum  Inputs=+-
  Subtract7 : Sum  Inputs=+-
  PIOut : Outport
  wires:
  Iq/1 -> Subtract7/1
  Id/1 -> Subtract6/1
  Constant8/1 -> ?
  Product3/1 -> Add/1
  Subtract6/1 -> Product3/1
  Product5/1 -> Add/2
  Iq_e/1 -> Subtract7/2, Product5/2
  Subtract7/1 -> Product5/1
  Id_e/1 -> Product3/2, Subtract6/2
  PID Controller/1 -> Saturation/1
  Constant2/1 -> PID Controller/2
  Abs/1 -> PID Controller/1
  Constant3/1 -> PID Controller/3
  Saturation/1 -> PIOut/1
  Add/1 -> Abs/1

== system MtrCtrl_24V/Subsystem8/Subsystem7 ==
  Id : Inport
  Iq : Inport  Port=2
  Id_e : Inport  Port=3
  Iq_e : Inport  Port=4
  Ud : Inport  Port=5
  Uq : Inport  Port=6
  Abs : Abs  SaturateOnIntegerOverflow=off
  Add : Sum
  Constant2 : Constant  Value=0.5
  Constant3 : Constant  Value=0.002
  Constant8 : Constant  Commented=on  Value=1/2/Ls
  Delay : Delay  DelayLength=1
  Delay1 : Delay  DelayLength=1
  PID Controller : slpidlib/PID Controller  Controller=PI  Form=Parallel  TimeDomain=Discrete-time  UseExternalTs=off  SampleTime=-1  IntegratorMethod=Forward Euler  FilterMethod=Forward Euler  ControllerParametersSource=external  P=1  I=1  UseKiTs=off  D=0  N=100  UseFilter=on  TunerSelectOption=Transfer Function Based (PID Tuner App)  InitialConditionSource=internal  InitialConditionForIntegrator=0  InitialConditionForFilter=0  DifferentiatorICPrevScaledInput=0  ExternalReset=none  TrackingMode=off  Kt=1  LimitOutput=off  SatLimitsSource=internal  UpperSaturationLimit=inf  LowerSaturationLimit=-inf  LinearizeAsGain=on  AntiWindupMode=none  Kb=1  LimitIntegrator=off  UpperIntegratorSaturationLimit=inf  LowerIntegratorSaturationLimit=-inf  POutMin=[]  POutMax=[]  IOutMin=[]  IOutMax=[]  DOutMin=[]  DOutMax=[]  NOutMin=[]  NOutMax=[]  SumOutMin=[]  SumOutMax=[]  SaturationOutMin=[]  SaturationOutMax=[]  PParamMin=[]  PParamMax=[]  IParamMin=[]  IParamMax=[]  DParamMin=[]  DParamMax=[]  NParamMin=[]  NParamMax=[]  KbParamMin=[]  KbParamMax=[]  KtParamMin=[]  KtParamMax=[]  KbOutMin=[]  KbOutMax=[]  KtOutMin=[]  KtOutMax=[]  IntegratorOutMin=[]  IntegratorOutMax=[]  FilterOutMin=[]  FilterOutMax=[]  SumI1OutMin=[]  SumI1OutMax=[]  SumI2OutMin=[]  SumI2OutMax=[]  SumI3OutMin=[]  SumI3OutMax=[]  SumI4OutMin=[]  SumI4OutMax=[]  SumDOutMin=[]  SumDOutMax=[]  DifferentiatorOutMin=[]  DifferentiatorOutMax=[]  FilterDiffOutCoefMin=[]  FilterDiffOutCoefMax=[]  ReciprocalOutMin=[]  ReciprocalOutMax=[]  SumDenOutMin=[]  SumDenOutMax=[]  SumNumOutMin=[]  SumNumOutMax=[]  DivideOutMin=[]  DivideOutMax=[]  UdiffTsProdOutMin=[]  UdiffTsProdOutMax=[]  NTsProdOutMin=[]  NTsProdOutMax=[]  UintegralTsProdOutMin=[]  UintegralTsProdOutMax=[]  UngainTsProdOutMin=[]  UngainTsProdOutMax=[]  ClampingZeroOutDataTypeStr=Inherit: Inherit via back propagation  ClampingZeroOutMin=[]  ClampingZeroOutMax=[]  FilterDenConstantOutDataTypeStr=Inherit: Inherit via back propagation  FilterDenConstantOutMin=[]  FilterDenConstantOutMax=[]  PCopyOutDataTypeStr=Inherit: Inherit via back propagation  PCopyOutMin=[]  PCopyOutMax=[]  NCopyOutDataTypeStr=Inherit: Inherit via back propagation  NCopyOutMin=[]  NCopyOutMax=[]  IntegratorContinuousStateAttributes=''  IntegratorStateMustResolveToSignalObject=off  IntegratorRTWStateStorageClass=Auto  FilterContinuousStateAttributes=''  FilterStateMustResolveToSignalObject=off  FilterRTWStateStorageClass=Auto  ParallelPVariant=ExternalParameters  IdealPVariant=Disabled  IVariant=ExternalParameters  DVariant=Disabled  IntegratorVariant=Discrete  SatVariant=Disabled  AWVariant=Passthrough  PCopyVariant=Disabled  TRVariant=Disabled  FdbkBlocksVariant=Forward  IdealPFdbkVariant=Disabled  SatFdbkVariant=Disabled  DerivativeFilterVariant=Disabled  NVariant=Disabled  NCopyVariant=Disabled_SignalSpec  FilterICVariant=Disabled  IntegratorICVariant=InternalICs  ExternalResetVariant=Disabled  TRSumVariant=Passthrough  SumFdbkVariant=Disabled  SumVariant=Sum_PI  TsampFilterVariant=InternalTs  TsampNgainVariant=Passthrough  TsampIntegralVariant=Disabled_SignalSpec  ExternalSaturationOutDataTypeStr=Inherit: Same as second input
  Product3 : Product
  Product5 : Product
  Saturation1 : Saturate  UpperLimit=1e6  LowerLimit=0.1
  Scope : Scope
  Subtract{1..2,6..7} (4 alike) : Sum  Inputs=+-
  PIOut : Outport
  wires:
  Id_e/1 -> Subtract6/2
  Add/1 -> Abs/1
  Subtract7/1 -> Product5/1
  Iq_e/1 -> Subtract7/2
  Product5/1 -> Add/2
  Subtract6/1 -> Product3/1
  Product3/1 -> Add/1
  Constant8/1 -> ?
  Id/1 -> Subtract6/1
  PID Controller/1 -> Scope/1, Saturation1/1
  Iq/1 -> Subtract7/1
  Delay/1 -> Subtract1/2
  Ud/1 -> Delay/1, Subtract1/1
  Subtract1/1 -> Product3/2
  Delay1/1 -> Subtract2/2
  Uq/1 -> Delay1/1, Subtract2/1
  Subtract2/1 -> Product5/2
  Saturation1/1 -> PIOut/1
  Constant3/1 -> PID Controller/3
  Abs/1 -> PID Controller/1
  Constant2/1 -> PID Controller/2

== system MtrCtrl_24V/TqCtrl/Subsystem1 ==
  Ref : Inport
  Fbk : Inport  Port=2
  Sat : Inport  Port=3
  Add : Sum
  Add1 : Sum
  Add2 : Sum  Inputs=+-
  Gain : Gain  Gain=20
  Ki : Constant  Value=0.01
  Kp : Constant  Value=1/Kt
  Product : Product
  Product1 : Product
  Relational Operator : RelationalOperator  Operator=<=  OutDataTypeStr=boolean  RndMeth=Simplest  InputSameDT=off
  Saturation : Saturate  UpperLimit=120  LowerLimit=-130
  Switch : Switch  Criteria=u2 > Threshold  SaturateOnIntegerOverflow=off  InputSameDT=off
  Unit Delay : UnitDelay  SampleTime=-1  HasFrameUpgradeWarning=on
  PIOut : Outport
  wires:
  Kp/1 -> Product/2
  Add1/1 -> PIOut/1
  Product/1 -> Saturation/1
  Add2/1 -> Product1/2, Product/1
  Add/1 -> Switch/1, Relational Operator/1
  Ki/1 -> Product1/1
  Relational Operator/1 -> Switch/2
  Gain/1 -> Relational Operator/2, Switch/3
  Sat/1 -> Gain/1
  Switch/1 -> Add1/2, Unit Delay/1
  Ref/1 -> Add2/1
  Fbk/1 -> Add2/2
  Saturation/1 -> Add1/1
  Product1/1 -> Add/1
  Unit Delay/1 -> Add/2

== system MtrCtrl_24V/CurLpCtrl/CurPILp/Subsystem ==
  IqFb : Inport  OutDataTypeStr=fixdt(1,32,31)
  IdFb : Inport  Port=2  OutDataTypeStr=fixdt(1,32,31)
  wm : Inport  Port=3  OutDataTypeStr=fixdt(1,32,31)
  Enable : EnablePort
  Add : Sum  OutDataTypeStr=fixdt(1,32,31)
  Flux : Constant  Value=C_PMSM_Flux_u32n32_Vs  OutDataTypeStr=fixdt(0,32,32)
  Gain : Gain  Gain=C_PMSM_PolePairs_u8_Null  OutDataTypeStr=fixdt(1,32,31)
  Ld : Gain  Gain=C_PMSM_Ls_pu/4  OutDataTypeStr=fixdt(1,32,31)
  Lq : Gain  Gain=C_PMSM_Ls_pu/2  OutDataTypeStr=fixdt(1,32,31)
  Product : Product  OutDataTypeStr=fixdt(1,32,31)
  Product1 : Product  OutDataTypeStr=fixdt(1,32,31)
  Vdff : Outport
  Vqff : Outport  Port=2
  wires:
  IdFb/1 -> Ld/1
  wm/1 -> Gain/1
  Ld/1 -> Add/1
  Flux/1 -> Add/2
  Add/1 -> Product/1
  Product/1 -> Vqff/1
  IqFb/1 -> Lq/1
  Lq/1 -> Product1/1
  Gain/1 -> Product1/2, Product/2
  Product1/1 -> Vdff/1

== system MtrCtrl_24V/CurLpCtrl/CurPILp/Subsystem1 ==
  Ref : Inport  OutDataTypeStr=fixdt(1,32,31)
  Fbk : Inport  Port=2  OutDataTypeStr=fixdt(1,32,31)
  Sat : Inport  Port=3  OutDataTypeStr=fixdt(0,32,32)
  Add : Sum  OutDataTypeStr=fixdt(1,32,31)
  Add1 : Sum  OutDataTypeStr=fixdt(1,32,31)
  Add2 : Sum  Inputs=+-  OutDataTypeStr=fixdt(1,32,31)
  Constant : Constant  Value=K_CCM_MRASEna_bool_Flg
  Constant1 : Constant  Value=K_CCM_MRASEna_bool_Flg
  Data Store Read2 : DataStoreRead  DataStoreName=MRAS_Ki  IndexOptions=Index vector (dialog)  Indices=1  OutputSizes=1
  Data Store Read3 : DataStoreRead  DataStoreName=MRAS_Kp  IndexOptions=Index vector (dialog)  Indices=1  OutputSizes=1
  Gain : Gain  Gain=2/3  OutDataTypeStr=fixdt(0,32,32)
  Ki : Constant  Value=C_PMSM_CurQKi_u32n31_null  OutDataTypeStr=fixdt(0,32,21)
  Kp : Constant  Value=C_PMSM_CurQKp_u32n31_null
  Product : Product  OutDataTypeStr=fixdt(1,32,31)
  Product1 : Product  OutDataTypeStr=fixdt(1,32,31)
  Relational Operator : RelationalOperator  Operator=<=  OutDataTypeStr=boolean  RndMeth=Simplest  InputSameDT=off
  Relational Operator1 : RelationalOperator  Operator=<=  OutDataTypeStr=boolean  RndMeth=Simplest  InputSameDT=off
  Scope : Scope  NumInputPorts=2
  Switch : Switch  Criteria=u2 > Threshold  OutDataTypeStr=fixdt(1,32,31)  SaturateOnIntegerOverflow=off  InputSameDT=off
  Switch1 : Switch  Criteria=u2 > Threshold  OutDataTypeStr=fixdt(1,32,31)  SaturateOnIntegerOverflow=off  InputSameDT=off
  Switch2 : Switch  Criteria=u2 > Threshold  SaturateOnIntegerOverflow=off  InputSameDT=off
  Switch3 : Switch  Criteria=u2 > Threshold  SaturateOnIntegerOverflow=off  InputSameDT=off
  Unit Delay : UnitDelay  SampleTime=-1  HasFrameUpgradeWarning=on
  PIOut : Outport
  wires:
  Add1/1 -> PIOut/1
  Add2/1 -> Product/1, Product1/2
  Ref/1 -> Add2/1
  Fbk/1 -> Add2/2
  Product1/1 -> Add/1
  Unit Delay/1 -> Add/2
  Product/1 -> Switch1/1, Relational Operator1/1
  Relational Operator1/1 -> Switch1/2
  Relational Operator/1 -> Switch/2
  Gain/1 -> Switch/3, Switch1/3, Relational Operator1/2, Relational Operator/2
  Sat/1 -> Gain/1
  Switch/1 -> Scope/2, Unit Delay/1, Add1/2
  Switch1/1 -> Scope/1, Add1/1
  Add/1 -> Relational Operator/1, Switch/1
  Data Store Read3/1 -> Switch2/1
  Data Store Read2/1 -> Switch3/1
  Kp/1 -> Switch2/3
  Constant/1 -> Switch2/2
  Switch2/1 -> Product/2
  Ki/1 -> Switch3/3
  Constant1/1 -> Switch3/2
  Switch3/1 -> Product1/1

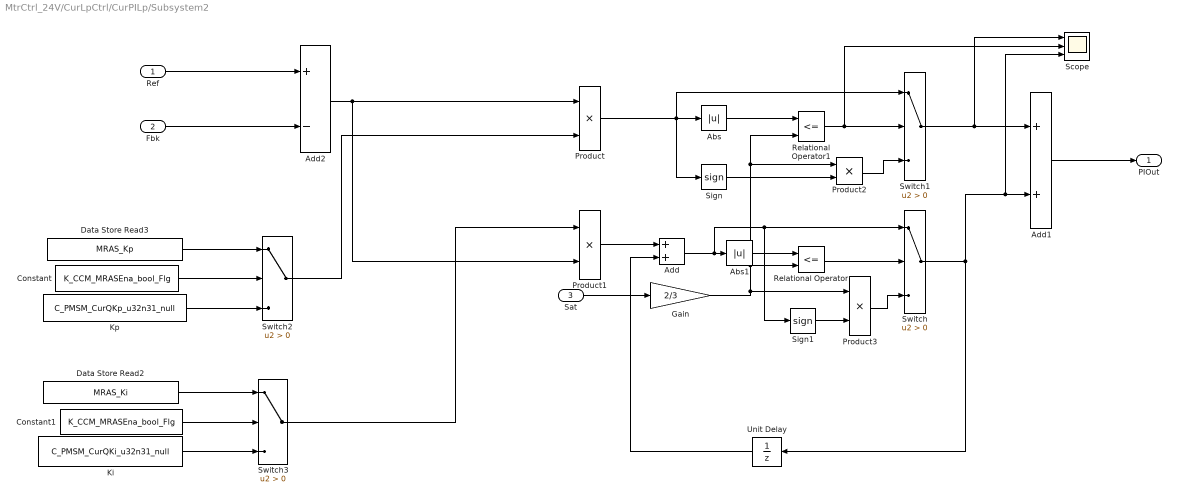
== system MtrCtrl_24V/CurLpCtrl/CurPILp/Subsystem2 ==
  Ref : Inport  OutDataTypeStr=fixdt(1,32,31)
  Fbk : Inport  Port=2  OutDataTypeStr=fixdt(1,32,31)
  Sat : Inport  Port=3  OutDataTypeStr=fixdt(0,32,32)
  Abs : Abs  SaturateOnIntegerOverflow=off
  Abs1 : Abs  SaturateOnIntegerOverflow=off
  Add : Sum  OutDataTypeStr=fixdt(1,32,31)
  Add1 : Sum  OutDataTypeStr=fixdt(1,32,31)
  Add2 : Sum  Inputs=+-  OutDataTypeStr=fixdt(1,32,31)
  Constant : Constant  Value=K_CCM_MRASEna_bool_Flg
  Constant1 : Constant  Value=K_CCM_MRASEna_bool_Flg
  Data Store Read2 : DataStoreRead  DataStoreName=MRAS_Ki  IndexOptions=Index vector (dialog)  Indices=1  OutputSizes=1
  Data Store Read3 : DataStoreRead  DataStoreName=MRAS_Kp  IndexOptions=Index vector (dialog)  Indices=1  OutputSizes=1
  Gain : Gain  Gain=2/3  OutDataTypeStr=fixdt(0,32,32)
  Ki : Constant  Value=C_PMSM_CurQKi_u32n31_null  OutDataTypeStr=fixdt(0,32,21)
  Kp : Constant  Value=C_PMSM_CurQKp_u32n31_null
  Product : Product  OutDataTypeStr=fixdt(1,32,31)
  Product1 : Product  OutDataTypeStr=fixdt(1,32,31)
  Product2 : Product
  Product3 : Product
  Relational Operator : RelationalOperator  Operator=<=  OutDataTypeStr=boolean  RndMeth=Simplest  InputSameDT=off
  Relational Operator1 : RelationalOperator  Operator=<=  OutDataTypeStr=boolean  RndMeth=Simplest  InputSameDT=off
  Scope : Scope  NumInputPorts=3
  Sign : Signum
  Sign1 : Signum
  Switch : Switch  Criteria=u2 > Threshold  OutDataTypeStr=fixdt(1,32,31)  SaturateOnIntegerOverflow=off  InputSameDT=off
  Switch1 : Switch  Criteria=u2 > Threshold  OutDataTypeStr=fixdt(1,32,31)  SaturateOnIntegerOverflow=off  InputSameDT=off
  Switch2 : Switch  Criteria=u2 > Threshold  SaturateOnIntegerOverflow=off  InputSameDT=off
  Switch3 : Switch  Criteria=u2 > Threshold  SaturateOnIntegerOverflow=off  InputSameDT=off
  Unit Delay : UnitDelay  SampleTime=-1  HasFrameUpgradeWarning=on
  PIOut : Outport
  wires:
  Add/1 -> Sign1/1, Switch/1, Abs1/1
  Switch1/1 -> Scope/1, Add1/1
  Switch/1 -> Scope/3, Add1/2, Unit Delay/1
  Sat/1 -> Gain/1
  Gain/1 -> Product3/1, Relational Operator/2, Relational Operator1/2, Product2/1
  Relational Operator/1 -> Switch/2
  Relational Operator1/1 -> Scope/2, Switch1/2
  Unit Delay/1 -> Add/2
  Product1/1 -> Add/1
  Fbk/1 -> Add2/2
  Ref/1 -> Add2/1
  Switch3/1 -> Product1/1
  Add1/1 -> PIOut/1
  Switch2/1 -> Product/2
  Add2/1 -> Product/1, Product1/2
  Product/1 -> Switch1/1, Sign/1, Abs/1
  Abs1/1 -> Relational Operator/1
  Abs/1 -> Relational Operator1/1
  Sign/1 -> Product2/2
  Product2/1 -> Switch1/3
  Sign1/1 -> Product3/2
  Product3/1 -> Switch/3
  Constant1/1 -> Switch3/2
  Kp/1 -> Switch2/3
  Constant/1 -> Switch2/2
  Data Store Read2/1 -> Switch3/1
  Ki/1 -> Switch3/3
  Data Store Read3/1 -> Switch2/1

== system MtrCtrl_24V/CurLpCtrl/CurPILp/Subsystem3 ==
  Vqcmd : Inport  OutDataTypeStr=fixdt(0,32,25)
  Constant6 : Constant  Value=OneOverUBase_V  OutDataTypeStr=fixdt(0,32,32)
  Product : Product  OutDataTypeStr=fixdt(1,32,31)
  Out1 : Outport
  wires:
  Vqcmd/1 -> Product/1
  Constant6/1 -> Product/2
  Product/1 -> Out1/1

== system MtrCtrl_24V/CurLpCtrl/SVPWM/Overmodulation ==
  Tx : Inport  OutDataTypeStr=fixdt(0,32,30)
  Ty : Inport  Port=2  OutDataTypeStr=fixdt(0,32,30)
  Add : Sum  OutDataTypeStr=fixdt(0,32,32)
  Chart : Stateflow chart  TreatAsAtomicUnit=on
  Constant : Constant  OutDataTypeStr=fixdt(0,32,31)
  Constant1 : Constant  Value=0.95  OutDataTypeStr=fixdt(0,32,32)
  Constant2 : Constant  Value=01  OutDataTypeStr=fixdt(0,32,31)
  Data Type Conversion : DataTypeConversion  SaturateOnIntegerOverflow=off  RndMeth=Floor
  Data Type Conversion1 : DataTypeConversion  SaturateOnIntegerOverflow=off  RndMeth=Floor
  Data Type Conversion2 : DataTypeConversion  SaturateOnIntegerOverflow=off  RndMeth=Floor
  Product2 : Product  OutDataTypeStr=fixdt(0,32,32)
  Scope : Scope  NumInputPorts=5
  Subsystem2 : Subsystem
  Switch : Switch  Criteria=u2 > Threshold  OutDataTypeStr=fixdt(0,32,33)  SaturateOnIntegerOverflow=off  InputSameDT=off
  Switch1 : Switch  Criteria=u2 > Threshold  OutDataTypeStr=fixdt(0,32,33)  SaturateOnIntegerOverflow=off  InputSameDT=off
  Tx_out : Outport
  Ty_out : Outport  Port=2
  wires:
  Constant1/1 -> Product2/2
  Constant/1 -> Product2/1
  Tx/1 -> Scope/2, Add/1, Chart/2(Ty), Subsystem2/2(Tx)
  Ty/1 -> Scope/3, Add/2, Chart/3(Tx), Subsystem2/3(Ty)
  Product2/1 -> Data Type Conversion2/1, Subsystem2/1(Ts)
  Subsystem2/1(Tx_o) -> Switch/1
  Chart/1(Tx_o) -> Data Type Conversion1/1
  Switch/1 -> Scope/4, Tx_out/1
  Switch1/1 -> Scope/5, Ty_out/1
  Subsystem2/2(Ty_o) -> Switch1/1
  Chart/2(Ty_o) -> Data Type Conversion/1
  Constant2/1 -> Switch1/2, Switch/2
  Add/1 -> Scope/1
  Data Type Conversion/1 -> Switch1/3
  Data Type Conversion1/1 -> Switch/3
  Data Type Conversion2/1 -> Chart/1(Ts)

== system MtrCtrl_24V/CurLpCtrl/SVPWM/Sector ==
  Alpha : Inport  OutDataTypeStr=fixdt(1,32,31)
  Beta : Inport  Port=2  OutDataTypeStr=fixdt(1,32,31)
  Add : Sum  Inputs=-+  OutDataTypeStr=fixdt(1,32,31)
  Add1 : Sum  Inputs=--  OutDataTypeStr=fixdt(1,32,31)
  Add2 : Sum  Inputs=3  OutDataTypeStr=fixdt(0,32,29)
  Chart : Stateflow chart  TreatAsAtomicUnit=on
  Compare To Constant : simulink/Logic and Bit Operations/Compare To Constant  relop=>  const=0  OutDataTypeStr=uint8
  Compare To Constant1 : simulink/Logic and Bit Operations/Compare To Constant  relop=>  const=0  OutDataTypeStr=uint8
  Compare To Constant2 : simulink/Logic and Bit Operations/Compare To Constant  relop=>  const=0  OutDataTypeStr=uint8
  Constant : Constant  Commented=on  Value=1/UBase_V
  Data Type Conversion : DataTypeConversion  SaturateOnIntegerOverflow=off  RndMeth=Floor
  Data Type Conversion1 : DataTypeConversion  SaturateOnIntegerOverflow=off  RndMeth=Floor
  Gain : Gain  Gain=2  OutDataTypeStr=fixdt(0,32,30)
  Gain1 : Gain  Gain=4  OutDataTypeStr=fixdt(0,32,29)
  Product : Product  Commented=on
  Product1 : Product  Commented=on
  Scope3 : Scope
  one_by_two : Gain  Gain=1/2  OutDataTypeStr=fixdt(1,32,31)  RndMeth=Simplest
  sqrt3_by_two : Gain  Gain=sqrt(3)/2  OutDataTypeStr=fixdt(1,32,31)  RndMeth=Simplest
  Sector : Outport
  Tx : Outport  Port=2
  Ty : Outport  Port=3
  wires:
  Add1/1 -> Compare To Constant2/1, Chart/3(Uc)
  Add/1 -> Compare To Constant1/1, Chart/2(Ub)
  one_by_two/1 -> Add1/1, Add/1
  sqrt3_by_two/1 -> Add1/2, Add/2
  Compare To Constant/1 -> Add2/1
  Compare To Constant1/1 -> Gain/1
  Compare To Constant2/1 -> Gain1/1
  Chart/1(Sector) -> Sector/1
  Gain/1 -> Add2/2
  Gain1/1 -> Add2/3
  Add2/1 -> Chart/4(N), Scope3/1  "N"
  Chart/2(Tx) -> Data Type Conversion/1
  Chart/3(Ty) -> Data Type Conversion1/1
  Beta/1 -> Chart/1(Ua), Compare To Constant/1, one_by_two/1
  Alpha/1 -> sqrt3_by_two/1
  Constant/1 -> Product1/2, Product/2
  Data Type Conversion/1 -> Tx/1
  Data Type Conversion1/1 -> Ty/1

== system MtrCtrl_24V/CurLpCtrl/SVPWM/SelectRegion ==
  V1 : Inport  OutDataTypeStr=fixdt(1,32,31)
  V2 : Inport  Port=2  OutDataTypeStr=fixdt(1,32,32)
  V3 : Inport  Port=3  OutDataTypeStr=fixdt(1,32,32)
  A : Switch  Criteria=u2 > Threshold  OutDataTypeStr=fixdt(0,32,30)  RndMeth=Zero  SaturateOnIntegerOverflow=off  InputSameDT=off
  B : Switch  Criteria=u2 > Threshold  OutDataTypeStr=fixdt(0,32,29)  RndMeth=Zero  SaturateOnIntegerOverflow=off  InputSameDT=off
  C : Switch  Criteria=u2 > Threshold  OutDataTypeStr=fixdt(0,32,30)  RndMeth=Zero  SaturateOnIntegerOverflow=off  InputSameDT=off
  Constant1 : Constant  OutDataTypeStr=fixdt(0,32,30)
  Constant2 : Constant  OutDataTypeStr=fixdt(0,32,30)
  Constant3 : Constant  Value=3  OutDataTypeStr=fixdt(0,32,30)
  Constant4 : Constant  Value=7  OutDataTypeStr=fixdt(0,32,29)
  Sum : Sum  Inputs=-+|  OutDataTypeStr=fixdt(0,32,30)
  Sum1 : Sum  Inputs=|-+  OutDataTypeStr=fixdt(0,32,29)  AccumDataTypeStr=fixdt(0,32,29)
  Sum2 : Sum  Inputs=-+|  OutDataTypeStr=fixdt(0,32,30)
  N : Outport
  wires:
  B/1 -> N/1
  V2/1 -> A/2
  Constant3/1 -> A/3, Sum/2
  Constant1/1 -> Sum/1
  Sum/1 -> A/1
  V3/1 -> C/2
  V1/1 -> B/2
  A/1 -> C/3, Sum2/2
  Constant2/1 -> Sum2/1
  Sum2/1 -> C/1
  C/1 -> B/1, Sum1/1
  Sum1/1 -> B/3
  Constant4/1 -> Sum1/2
